simulink model "KALM_filter_DTC_6Sector"  (R2018a)
settings: Solver=ode45  StartTime=0.0  StopTime=6  RelTol=1e-3
values from neighbouring files (symbols this model uses):
  Ah = [0 0 0 0;0 0 0 0;0 1/(Ls*segma) 0 -1;-1/(Ls*segma) 0 1 0]    [Untitled.m]
  Ak = [0 0 -Rs 0; 0 0 0 -Rs; 1/(Tr*Ls*segma) 0 -(1/Ts+1/Tr)/segma 0;     0 1/(Tr*Ls*segma) 0 -(1/Ts+1/Tr)/segma ]    [Untitled.m]
  B = [1 0 1/(Ls*segma) 0;0 1 0 1/(Ls*segma)]'    [Untitled.m]
  J = 0.031    [Untitled.m]
  p = 2    [Untitled.m]
undefined symbols (not defined in the file or in its folder): sigbuilder_block
libraries: powerlib x11, simulink_need_slupdate x1, re_lib x1, powerlib_meascontrol x1
settings Model: Creator=Dell  LastModifiedBy=Dell

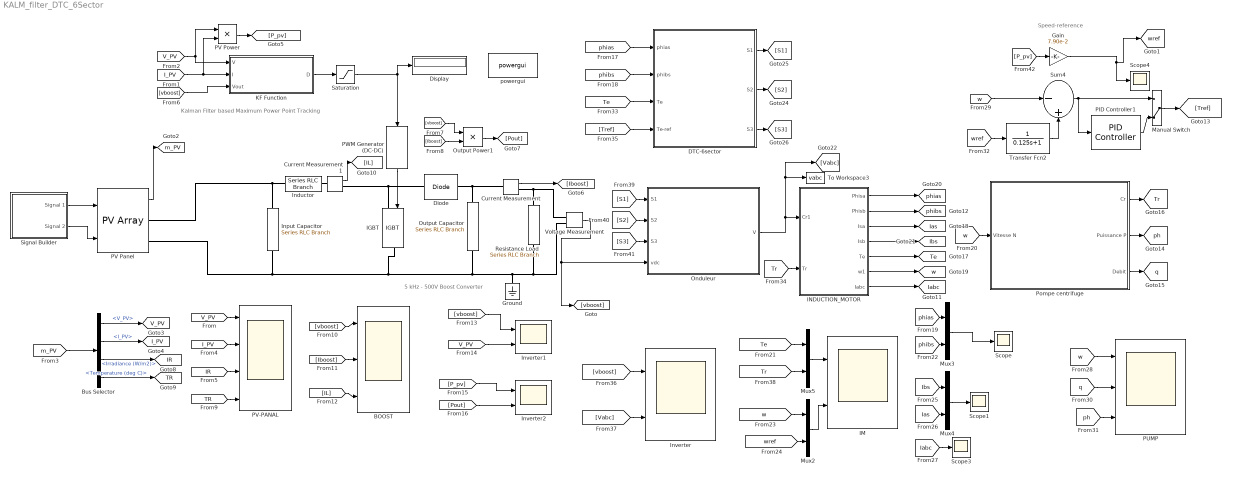
== system KALM_filter_DTC_6Sector ==
  note: 5 kHz - 500V
      | Boost Converter
  note: Kalman Filter based Maximum Power Point Tracking
  note: Speed-reference
  " Resistance Load      " : powerlib/Elements/Series RLC Branch  LConnTagsString=__new0  RConnTagsString=__new0  BranchType=R  Resistance=100  Inductance=1e-3  SetiL0=off  InitialCurrent=0  Capacitance=1e-6  Setx0=off  InitialVoltage=0  Measurements=None
  " Output Capacitor   " : powerlib/Elements/Series RLC Branch  LConnTagsString=__new0  RConnTagsString=__new0  BranchType=C  Resistance=1  Inductance=1e-3  SetiL0=off  InitialCurrent=0  Capacitance=100e-6  Setx0=off  InitialVoltage=0  Measurements=None
  BOOST : Scope  NumInputPorts=3
  Bus Selector : BusSelector  OutputSignals=V_PV,I_PV,Irradiance (W/m2),Temperature (deg C)
  Current Measurement : powerlib/Measurements/Current Measurement  PhasorSimulation=off  OutputType=Complex  PSBequivalent=0
  Current Measurement1 : powerlib/Measurements/Current Measurement  PhasorSimulation=off  OutputType=Complex  PSBequivalent=0
  DTC-6sector : Subsystem
  Diode : powerlib/Power Electronics/Diode  Ron=0.001  Lon=0  Vf=0.8  IC=0  UseSnubber=off  Rs=500  Cs=250e-9  Measurements=off
  Display : Display
  Gain : Gain  Gain=7.90e-2
  Ground : powerlib/Elements/Ground  LConnTagsString=a
  "IGBT  " : powerlib/Power Electronics/IGBT  Ron=0.001  Lon=0  Vf=1  Tf=1e-6  Tt=2e-6  IC=0  Rs=1e5  Cs=inf  Measurements=off
  IM : Scope  NumInputPorts=2
  INDUCTION_MOTOR : Subsystem  mask(Moteur Asynchrone){}
  "Inductor " : powerlib/Elements/Series RLC Branch  LConnTagsString=__new0  RConnTagsString=__new0  BranchType=L  Resistance=0.005  Inductance=3e-3  SetiL0=off  InitialCurrent=0  Capacitance=1e-6  Setx0=off  InitialVoltage=0  Measurements=None
  "Input Capacitor " : powerlib/Elements/Series RLC Branch  LConnTagsString=__new0  RConnTagsString=__new0  BranchType=C  Resistance=1  Inductance=1e-3  SetiL0=off  InitialCurrent=0  Capacitance=100e-6  Setx0=off  InitialVoltage=0  Measurements=None
  Inverter : Scope  NumInputPorts=2
  Inverter1 : Scope  NumInputPorts=2
  Inverter2 : Scope  NumInputPorts=2
  KF Function : MATLAB Function  TreatAsAtomicUnit=on
  Manual Switch : ManualSwitch  CurrentSetting=0
  Mux{2..5} (4 alike) : Mux  Inputs=2
  Onduleur : Subsystem
      mask Display: disp('Onduleur')
  Output Power1 : Product
  PID Controller1 : simulink_need_slupdate/PID Controller  P=4  I=35  D=0
      settings: SourceProductName=Simulink
  PUMP : Scope  NumInputPorts=3
  PV Panel : re_lib/Solar/PV Array  Npar=1  Nser=8  PlotType=array @ 25 deg.C & specified irradiances  S_vec="[800  900 1000   ]"  Temp_C_vec="[ 45 25  ]"  ModuleName=China Sunergy (Nanjing) SST235-60P  PlotWhenSelected=off  Pm=235.024  Ncell=60  Voc=36.8  Isc=8.54  Vm=29.6  Im=7.94  beta_Voc_pc=-0.37  alpha_Isc_pc=0.06  beta_Voc=-0.13616  alpha_Isc=0.005124  IL=8.5548  I0=4.0556e-10  nI=1.0052  Rsh=194.4803  Rs=0.33595  BAL=off  Tc=1e-6  Tfilter=1e-5
      settings: AttributesFormatString=|
      | %<ModuleName>
      | %<Nser>-module string
      | %<Npar> parallel strings
  PV Power : Product
  PV-PANAL : Scope  NumInputPorts=4
  PWM Generator (DC-DC) : powerlib_meascontrol/Pulse & Signal Generators/PWM Generator (DC-DC)  Fsw=5000  Ts=1e-6
  Pompe centrifuge : Subsystem
  "Saturation " : Saturate  UpperLimit=1  LowerLimit=0
  Scope{,1,3..4} (4 alike) : Scope
  Signal Builder : Subsystem  Tag=STV Subsys  LoadFcn=sigbuilder_block('load');  StartFcn=sigbuilder_block('start');  StopFcn=sigbuilder_block('stop');  ClipboardFcn=sigbuilder_block('clipboard');  mask(Sigbuilder block){tuvar=[0:10]}
      mask help: Simulink:masks:SigbuilderBlock_MD
      mask init:
      | if ~strcmp(get_param(bdroot(gcbh),'SimulationStatus'),'stopped') tuvar = sigbuilder_block('maskInit'); end
      settings: CopyFcn=sigbuilder_block('copy');  DeleteFcn=sigbuilder_block('delete');  ModelCloseFcn=sigbuilder_block('modelClose');  PreSaveFcn=sigbuilder_block('preSave');  PauseFcn=sigbuilder_block('pause');  ContinueFcn=sigbuilder_block('continue');  NameChangeFcn=sigbuilder_block('namechange');  OpenFcn=sigbuilder_block('open',[257.25 132.75 550.5 359.25 ]);  CloseFcn=sigbuilder_block('close');
      mask Display: plot(0, 0, 100, 100,[2, 2, 32, 32, 2], [68, 8, 8, 68, 68],[32, 2], [38, 38], [32, 19, 2],[53, 60, 44], [32, 17, 17, 2],[16, 16, 31, 31]);txt = getActiveGroup(gcbh);text(2, 100, txt,'verticalAlignment', 'top');
  Sum4 : Sum  Inputs=|-+  SampleTime=0.00001
  To Workspace3 : ToWorkspace  VariableName=vabc  SampleTime=-1
  Transfer Fcn2 : TransferFcn  Denominator=[0.125 1]
  Voltage Measurement : powerlib/Measurements/Voltage Measurement  PhasorSimulation=off  OutputType=Complex  PSBequivalent=0
  powergui : powerlib/powergui  Priority=1  SimulationMode=Discrete  SampleTime=1e-6  frequency=60  Iterations=50  frequencyindice=0  Pbase=100e6  ErrMax=1e-4  UnitsV=kV  UnitsW=MW  buscounter=0  FunctionMessages=off  echomessages=off  EnableUseOfTLC=off  CurrentSourceSwitches=off  DisableSnubberDevices=off  DisableRonSwitches=off  DisableVfSwitches=off  DisplayEquations=off  SolverType=Tustin/Backward Euler (TBE)  Interpol=off  ExternalGateDelay=off  methode=off  Ts=100  x0status=blocks  SPID=on  SwTol=0  HookPort=off  RestoreLinks=warning  ResistiveCurrentMeasurement=off  Frange=[0:2:500]  Ylog=off  Xlog=on  ShowGrid=off  save=off  variable=ZData  structure=0  ZoomFFT=off  StartTime=0.0  cycles=1  DisplayStyle=1  fundamental=60  FreqAxis=off  MaxFrequency=1000  frequencyindicesteady=1  RmsSteady=1  display=off
  tag scope: IR=global, I_PV=global, Iabc=global, Ias=global, Ibs=global, TR=global, Te=global, Tr=global, V_PV=global, m_PV=global, ph=global, phias=global, phibs=global, q=global, w=global, wref=global
  wires:
  [w] -> PUMP/1
  [IL] -> BOOST/3
  [q] -> PUMP/2
  [w] -> Sum4/1
  [vboost] -> Inverter1/1
  Mux4/1 -> Scope1/1
  [S1] -> Onduleur/1(S1)
  "Saturation "/1 -> Display/1, PWM Generator (DC-DC)/1
  [S3] -> Onduleur/3(S3)
  [phibs] -> DTC-6sector/2(phibs)
  [ph] -> PUMP/3
  [Ias] -> Mux4/2
  DTC-6sector/1(S1) -> [S1]
  INDUCTION_MOTOR/7(Iabc) -> [Iabc]
  Current Measurement1/1 -> [IL]
  Mux5/1 -> IM/1
  [V_PV] -> PV Power/1, KF Function/1(V)
  Signal Builder/1(Signal 1) -> PV Panel/1
  [S2] -> Onduleur/2(S2)
  Bus Selector/1 -> [V_PV]  "<V_PV>"
  INDUCTION_MOTOR/5(Te) -> [Te]
  Pompe centrifuge/3(Debit) -> [q]
  [Pout] -> Inverter2/2
  [Te] -> Mux5/1
  INDUCTION_MOTOR/6(w1) -> [w]
  [Te] -> DTC-6sector/3(Te)
  [w] -> Pompe centrifuge/1(Vitesse N)
  [wref] -> Mux2/2
  [vboost] -> Inverter/1
  Sum4/1 -> Manual Switch/1, PID Controller1/1
  Signal Builder/2(Signal 2) -> PV Panel/2
  [phias] -> DTC-6sector/1(phias)
  [phias] -> Mux3/1
  Manual Switch/1 -> [Tref]
  [w] -> Mux2/1
  [Vabc] -> Inverter/2
  [Tr] -> Mux5/2
  INDUCTION_MOTOR/1(Phisa) -> [phias]
  [Tref] -> DTC-6sector/4(Te-ref)
  [Ibs] -> Mux4/1
  [vboost] -> KF Function/3(Vout)
  [m_PV] -> Bus Selector/1
  Bus Selector/3 -> [IR]  "<Irradiance (W/m2)>"
  [vboost] -> BOOST/1
  [V_PV] -> Inverter1/2
  Bus Selector/4 -> [TR]  "<Temperature (deg C)>"
  [phibs] -> Mux3/2
  [Iboost] -> BOOST/2
  INDUCTION_MOTOR/3(Isa) -> [Ias]
  [vboost] -> Output Power1/1
  PV Power/1 -> [P_pv]
  PWM Generator (DC-DC)/1 -> "IGBT  "/1
  Mux2/1 -> IM/2
  Output Power1/1 -> [Pout]
  DTC-6sector/3(S3) -> [S3]
  [Iboost] -> Output Power1/2
  KF Function/1(D) -> "Saturation "/1
  INDUCTION_MOTOR/2(Phisb) -> [phibs]
  [I_PV] -> PV-PANAL/2
  Voltage Measurement/1 -> Onduleur/4(vdc), [vboost]
  [P_pv] -> Inverter2/1
  Mux3/1 -> Scope/1
  [TR] -> PV-PANAL/4
  [Iabc] -> Scope3/1
  Pompe centrifuge/1(Cr) -> [Tr]
  [Tr] -> INDUCTION_MOTOR/2(Tr)
  Transfer Fcn2/1 -> Sum4/2
  PV Panel/1 -> [m_PV]
  DTC-6sector/2(S2) -> [S2]
  Bus Selector/2 -> [I_PV]  "<I_PV>"
  Pompe centrifuge/2("Puissance P ") -> [ph]
  INDUCTION_MOTOR/4(Isb) -> [Ibs]
  [wref] -> Transfer Fcn2/1
  Onduleur/1(V) -> INDUCTION_MOTOR/1(Cr1), [Vabc], To Workspace3/1
  [V_PV] -> PV-PANAL/1
  [IR] -> PV-PANAL/3
  Current Measurement/1 -> [Iboost]
  PID Controller1/1 -> Manual Switch/2
  [I_PV] -> PV Power/2, KF Function/2(I)
  [P_pv] -> Gain/1
  Gain/1 -> Scope4/1, [wref]
  connections:
  Ground/LConn1 -- PV Panel/RConn2 -- "Input Capacitor "/RConn1 -- "IGBT  "/RConn1 -- " Output Capacitor   "/RConn1 -- " Resistance Load      "/RConn1 -- Voltage Measurement/LConn2
  " Output Capacitor   "/LConn1 -- Diode/RConn1 -- Current Measurement/LConn1
  "Input Capacitor "/LConn1 -- PV Panel/RConn1 -- "Inductor "/LConn1
  "IGBT  "/LConn1 -- Diode/LConn1 -- Current Measurement1/RConn1
  " Resistance Load      "/LConn1 -- Current Measurement/RConn1 -- Voltage Measurement/LConn1
  Current Measurement1/LConn1 -- "Inductor "/RConn1

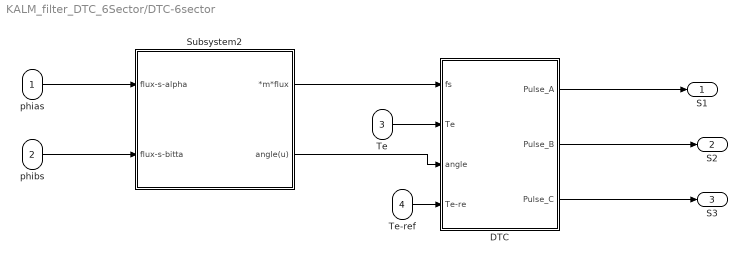
== system KALM_filter_DTC_6Sector/DTC-6sector ==
  phias : Inport
  phibs : Inport  Port=2
  Te : Inport  Port=3
  Te-ref : Inport  Port=4
  DTC : Subsystem
  Subsystem2 : Subsystem
  S1 : Outport
  S2 : Outport  Port=2
  S3 : Outport  Port=3
  wires:
  Te/1 -> DTC/2(Te)
  Subsystem2/1(*m*flux) -> DTC/1(fs)
  DTC/2(Pulse_B) -> S2/1
  Subsystem2/2(angle(u)) -> DTC/3(angle)
  DTC/1(Pulse_A) -> S1/1
  Te-ref/1 -> DTC/4(Te-re)
  DTC/3(Pulse_C) -> S3/1
  phibs/1 -> Subsystem2/2(flux-s-bitta)
  phias/1 -> Subsystem2/1(flux-s-alpha)

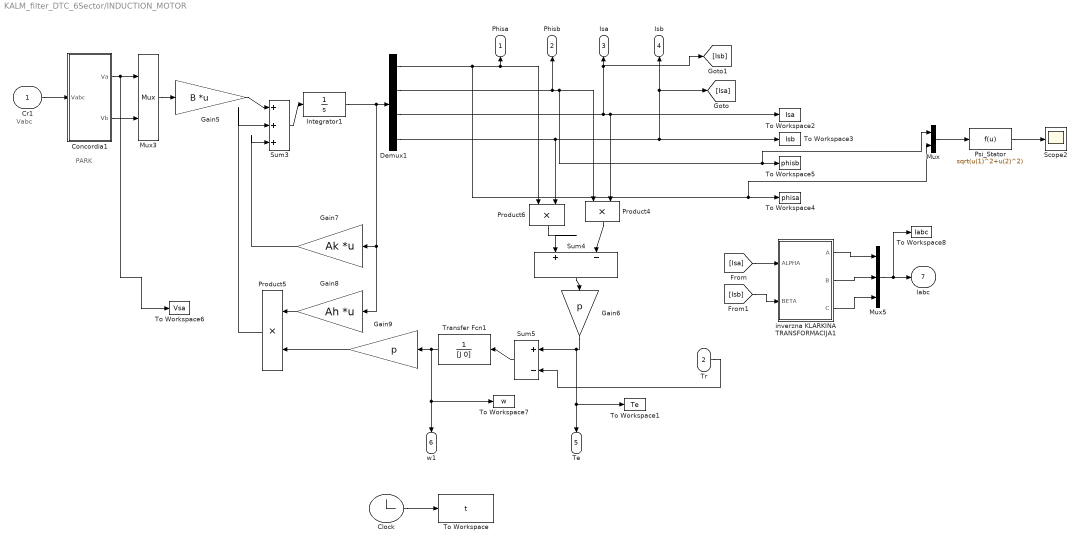
== system KALM_filter_DTC_6Sector/INDUCTION_MOTOR ==
  note: Vabc
  note: PARK
  Cr1 : Inport
  Tr : Inport  Port=2
  Clock : Clock
  Concordia1 : Subsystem
  Demux1 : Demux
  Gain5 : Gain  Gain=B  Multiplication=Matrix(K*u) (u vector)  SampleTime=0.00001
  Gain6 : Gain  Gain=p  SampleTime=0.00001
  Gain7 : Gain  Gain=Ak  Multiplication=Matrix(K*u)  SampleTime=0.00001
  Gain8 : Gain  Gain=Ah  Multiplication=Matrix(K*u)  SampleTime=0.00001
  Gain9 : Gain  Gain=p  SampleTime=0.00001
  Integrator1 : Integrator
  Mux : Mux  Inputs=2
  Mux3 : Mux  Inputs=2
  Mux5 : Mux  Inputs=3
  Product4 : Product  SampleTime=0.00001  RndMeth=Zero
  Product5 : Product  SampleTime=0.00001  RndMeth=Zero
  Product6 : Product  SampleTime=0.00001  RndMeth=Zero
  Psi_Stator : Fcn  Expr=sqrt(u(1)^2+u(2)^2)
  Scope2 : Scope
  Sum3 : Sum  Inputs=|+++  SampleTime=0.00001
  Sum4 : Sum  Inputs=|+-  SampleTime=0.00001
  Sum5 : Sum  Inputs=|+-  SampleTime=0.00001
  To Workspace : ToWorkspace  VariableName=t  SampleTime=0.00001
  To Workspace1 : ToWorkspace  VariableName=Te  SampleTime=-1
  To Workspace2 : ToWorkspace  VariableName=Isa  SampleTime=-1
  To Workspace3 : ToWorkspace  VariableName=Isb  SampleTime=-1
  To Workspace4 : ToWorkspace  VariableName=phisa  SampleTime=-1
  To Workspace5 : ToWorkspace  VariableName=phisb  SampleTime=-1
  To Workspace6 : ToWorkspace  VariableName=Vsa  SampleTime=-1
  To Workspace7 : ToWorkspace  VariableName=w  SampleTime=-1
  To Workspace8 : ToWorkspace  VariableName=Iabc  SampleTime=-1
  Transfer Fcn1 : TransferFcn  Denominator=[J 0]
  inverzna KLARKINA TRANSFORMACIJA1 : Subsystem
  Phisa : Outport
  Phisb : Outport  Port=2
  Isa : Outport  Port=3
  Isb : Outport  Port=4
  Te : Outport  Port=5
  w1 : Outport  Port=6
  Iabc : Outport  Port=7
  wires:
  Gain5/1 -> Sum3/1
  Sum5/1 -> Transfer Fcn1/1
  Gain8/1 -> Product5/1
  Sum3/1 -> Integrator1/1
  Integrator1/1 -> Demux1/1, Gain8/1, Gain7/1
  Clock/1 -> To Workspace/1
  Mux3/1 -> Gain5/1
  Transfer Fcn1/1 -> Gain9/1, w1/1, To Workspace7/1
  Demux1/3 -> Product4/2, To Workspace2/1, [Isb], Isa/1
  Demux1/4 -> Product6/2, Isb/1, [Isa], To Workspace3/1
  Gain6/1 -> Sum5/1, Te/1, To Workspace1/1
  Sum4/1 -> Gain6/1
  Product5/1 -> Sum3/2
  Gain7/1 -> Sum3/3
  Concordia1/2(Vb) -> Mux3/2
  Concordia1/1(Va) -> Mux3/1, To Workspace6/1
  Cr1/1 -> Concordia1/1(Vabc)
  Gain9/1 -> Product5/2
  Product6/1 -> Sum4/1
  Product4/1 -> Sum4/2
  inverzna KLARKINA TRANSFORMACIJA1/1(A) -> Mux5/1
  inverzna KLARKINA TRANSFORMACIJA1/2(B) -> Mux5/2
  Mux5/1 -> To Workspace8/1, Iabc/1
  [Isa] -> inverzna KLARKINA TRANSFORMACIJA1/1(ALPHA)
  [Isb] -> inverzna KLARKINA TRANSFORMACIJA1/2(BETA)
  inverzna KLARKINA TRANSFORMACIJA1/3(C) -> Mux5/3
  Tr/1 -> Sum5/2
  Psi_Stator/1 -> Scope2/1
  Demux1/1 -> Phisa/1, Product6/1, Mux/2, To Workspace4/1
  Mux/1 -> Psi_Stator/1
  Demux1/2 -> Phisb/1, Product4/1, Mux/1, To Workspace5/1

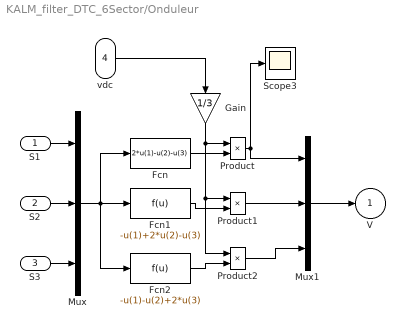
== system KALM_filter_DTC_6Sector/Onduleur ==
  S1 : Inport
  S2 : Inport  Port=2
  S3 : Inport  Port=3
  vdc : Inport  Port=4
  Fcn : Fcn  Expr=2*u(1)-u(2)-u(3)
  Fcn1 : Fcn  Expr=-u(1)+2*u(2)-u(3)
  Fcn2 : Fcn  Expr=-u(1)-u(2)+2*u(3)
  Gain : Gain  Gain=1/3  SaturateOnIntegerOverflow=on  OutDataTypeStr=Inherit: Same as input  ParamDataTypeStr=Inherit: Same as input
  Mux : Mux  Inputs=3
  Mux1 : Mux  Inputs=3
  Product : Product  SaturateOnIntegerOverflow=on  OutDataTypeStr=Inherit: Same as first input
  Product1 : Product  SaturateOnIntegerOverflow=on  OutDataTypeStr=Inherit: Same as first input
  Product2 : Product  SaturateOnIntegerOverflow=on  OutDataTypeStr=Inherit: Same as first input
  Scope3 : Scope
  V : Outport
  wires:
  Product2/1 -> Mux1/3
  Product1/1 -> Mux1/2
  Product/1 -> Mux1/1, Scope3/1
  Gain/1 -> Product2/1, Product1/1, Product/1
  vdc/1 -> Gain/1
  Fcn2/1 -> Product2/2
  Fcn1/1 -> Product1/2
  Fcn/1 -> Product/2
  Mux/1 -> Fcn1/1, Fcn2/1, Fcn/1
  S1/1 -> Mux/1
  S2/1 -> Mux/2
  S3/1 -> Mux/3
  Mux1/1 -> V/1

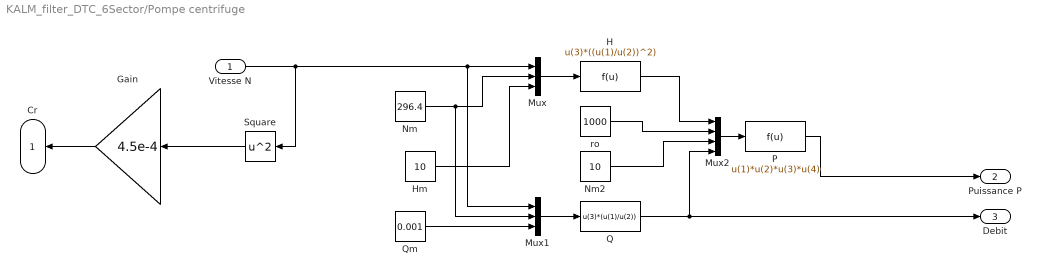
== system KALM_filter_DTC_6Sector/Pompe centrifuge ==
  Vitesse N : Inport
  Gain : Gain  Gain=4.5e-4
  H : Fcn  Expr=u(3)*((u(1)/u(2))^2)
  Hm : Constant  Value=10
  Mux : Mux  Inputs=3
  Mux1 : Mux  Inputs=3
  Mux2 : Mux
  Nm : Constant  Value=296.4
  Nm2 : Constant  Value=10
  "P " : Fcn  Expr=u(1)*u(2)*u(3)*u(4)
  Q : Fcn  Expr=u(3)*(u(1)/u(2))
  Qm : Constant  Value=0.001
  Square : Math  Operator=square  RndMeth=Zero  SaturateOnIntegerOverflow=on
  ro : Constant  Value=1000
  Cr : Outport
  "Puissance P " : Outport  Port=2
  Debit : Outport  Port=3
  wires:
  Square/1 -> Gain/1
  Gain/1 -> Cr/1
  "P "/1 -> "Puissance P "/1
  ro/1 -> Mux2/2
  Qm/1 -> Mux1/3
  Q/1 -> Debit/1, Mux2/4
  Mux2/1 -> "P "/1
  Mux/1 -> H/1
  Nm2/1 -> Mux2/3
  Mux1/1 -> Q/1
  Vitesse N/1 -> Square/1, Mux1/1, Mux/1
  H/1 -> Mux2/1
  Hm/1 -> Mux/3
  Nm/1 -> Mux1/2, Mux/2

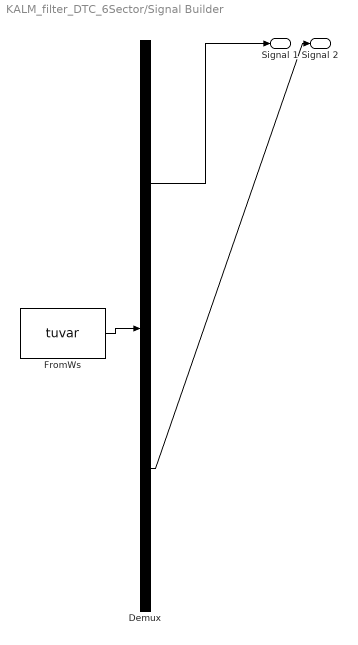
== system KALM_filter_DTC_6Sector/Signal Builder ==
  Demux : Demux  Tag=STV Demux  Outputs=2
  FromWs : FromWorkspace  Tag=STV FromWs  VariableName=tuvar  SampleTime=0
      SigBuilderData=|
      | common.afterFinalStr = 'Extrapolate'
      | common.sampleTime = 0
      | dataSet.timeRange = [0 6]
      | dataSet.name = 'Group 1'
      | sbobj.Groups.Name = 'Group 1'
      | sbobj.Groups.Signals(1).Name = 'Signal 1'
      | sbobj.Groups.Signals(1).XData = [0 1 1 2 2 3 3 4 4 5 5 6]
      | sbobj.Groups.Signals(1).YData = [600 600 800 800 1000 1000 805 800 700 700 600 600]
      | sbobj.Groups.Signals(2).Name = 'Signal 2'
      | sbobj.Groups.Signals(2).XData = [0 6]
      | sbobj.Groups.Signals(2).YData = [25 25]
      | sbobj.Groups.TimeRange = [0 6]
  Signal 1 : Outport  Tag=STV Outport
  Signal 2 : Outport  Tag=STV Outport  Port=2
  wires:
  Demux/1 -> Signal 1/1
  FromWs/1 -> Demux/1
  Demux/2 -> Signal 2/1

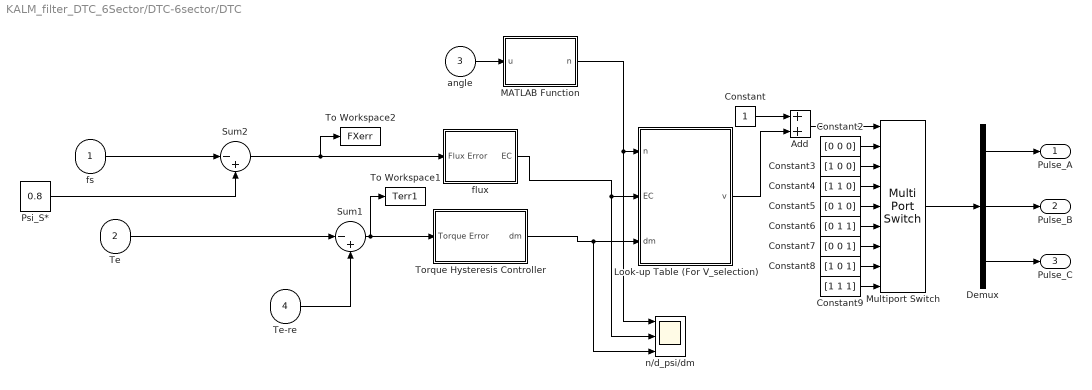
== system KALM_filter_DTC_6Sector/DTC-6sector/DTC ==
  fs : Inport
  Te : Inport  Port=2
  angle : Inport  Port=3
  Te-re : Inport  Port=4
  Add : Sum
  Constant : Constant
  Constant2 : Constant  Value=[0 0 0]
  Constant3 : Constant  Value=[1 0 0]
  Constant4 : Constant  Value=[1 1 0]
  Constant5 : Constant  Value=[0 1 0]
  Constant6 : Constant  Value=[0 1 1]
  Constant7 : Constant  Value=[0 0 1]
  Constant8 : Constant  Value=[1 0 1]
  Constant9 : Constant  Value=[1 1 1]
  Demux : Demux  Outputs=3
  Look-up Table (For V_selection) : MATLAB Function  TreatAsAtomicUnit=on
  MATLAB Function : MATLAB Function  TreatAsAtomicUnit=on
  Multiport Switch : MultiPortSwitch  Inputs=8
  Psi_S* : Constant  Value=0.8
  Sum1 : Sum  Inputs=|-+
  Sum2 : Sum  Inputs=|-+
  To Workspace1 : ToWorkspace  VariableName=Terr1  SampleTime=-1
  To Workspace2 : ToWorkspace  VariableName=FXerr  SampleTime=-1
  Torque Hysteresis Controller : Subsystem
  flux : Subsystem
  n/d_psi/dm : Scope  NumInputPorts=3
  Pulse_A : Outport
  Pulse_B : Outport  Port=2
  Pulse_C : Outport  Port=3
  wires:
  fs/1 -> Sum2/1
  MATLAB Function/1(n) -> Look-up Table (For V_selection)/1(n), n/d_psi/dm/1
  Torque Hysteresis Controller/1(dm) -> Look-up Table (For V_selection)/3(dm), n/d_psi/dm/3
  Psi_S*/1 -> Sum2/2
  Add/1 -> Multiport Switch/1
  Te/1 -> Sum1/1
  Constant9/1 -> Multiport Switch/9
  Constant6/1 -> Multiport Switch/6
  Constant2/1 -> Multiport Switch/2
  Constant3/1 -> Multiport Switch/3
  Constant5/1 -> Multiport Switch/5
  Demux/3 -> Pulse_C/1
  Constant8/1 -> Multiport Switch/8
  Look-up Table (For V_selection)/1(v) -> Add/2
  Constant/1 -> Add/1
  Demux/1 -> Pulse_A/1
  Demux/2 -> Pulse_B/1
  Constant7/1 -> Multiport Switch/7
  Constant4/1 -> Multiport Switch/4
  Multiport Switch/1 -> Demux/1
  flux/1(EC) -> Look-up Table (For V_selection)/2(EC), n/d_psi/dm/2
  Sum2/1 -> To Workspace2/1, flux/1(Flux Error)
  angle/1 -> MATLAB Function/1(u)
  Sum1/1 -> To Workspace1/1, Torque Hysteresis Controller/1(Torque Error)
  Te-re/1 -> Sum1/2

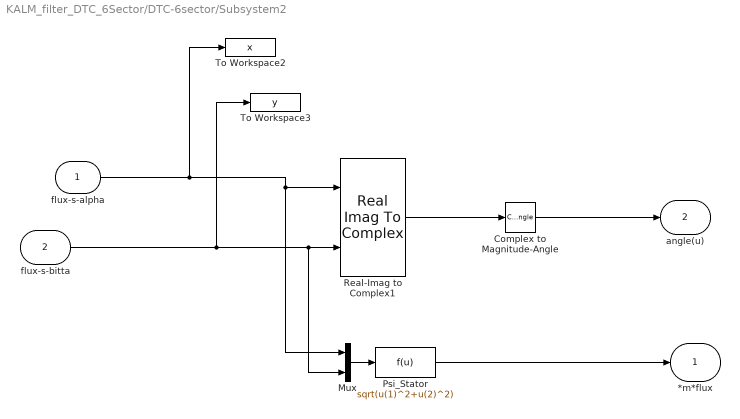
== system KALM_filter_DTC_6Sector/DTC-6sector/Subsystem2 ==
  flux-s-alpha : Inport
  flux-s-bitta : Inport  Port=2
  Complex to Magnitude-Angle : ComplexToMagnitudeAngle  Output=Angle
  Mux : Mux  Inputs=2
  Psi_Stator : Fcn  Expr=sqrt(u(1)^2+u(2)^2)
  Real-Imag to Complex1 : RealImagToComplex  SampleTime=0.00001
  To Workspace2 : ToWorkspace  VariableName=x  SampleTime=-1
  To Workspace3 : ToWorkspace  VariableName=y  SampleTime=-1
  *m*flux : Outport
  angle(u) : Outport  Port=2
  wires:
  Real-Imag to Complex1/1 -> Complex to Magnitude-Angle/1
  Complex to Magnitude-Angle/1 -> angle(u)/1
  Mux/1 -> Psi_Stator/1
  Psi_Stator/1 -> *m*flux/1
  flux-s-alpha/1 -> To Workspace2/1, Mux/1, Real-Imag to Complex1/1
  flux-s-bitta/1 -> Mux/2, Real-Imag to Complex1/2, To Workspace3/1

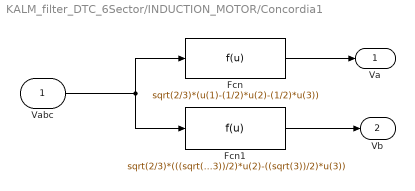
== system KALM_filter_DTC_6Sector/INDUCTION_MOTOR/Concordia1 ==
  Vabc : Inport
  Fcn : Fcn  Expr=sqrt(2/3)*(u(1)-(1/2)*u(2)-(1/2)*u(3))  SampleTime=0.00001
  Fcn1 : Fcn  Expr=sqrt(2/3)*(((sqrt(3))/2)*u(2)-((sqrt(3))/2)*u(3))  SampleTime=0.00001
  Va : Outport
  Vb : Outport  Port=2
  wires:
  Fcn/1 -> Va/1
  Fcn1/1 -> Vb/1
  Vabc/1 -> Fcn/1, Fcn1/1

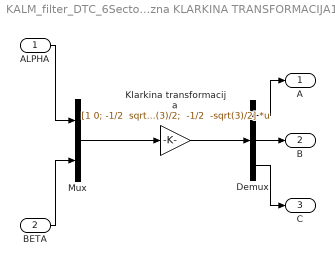
== system KALM_filter_DTC_6Sector/INDUCTION_MOTOR/inverzna KLARKINA TRANSFORMACIJA1 ==
  ALPHA : Inport
  BETA : Inport  Port=2
  Demux : Demux  Outputs=3
  Klarkina transformacija : Gain  Gain="[1 0; -1/2  sqrt(3)/2;  -1/2  -sqrt(3)/2]"  Multiplication=Matrix(K*u)
  Mux : Mux  Inputs=2
  A : Outport
  B : Outport  Port=2
  C : Outport  Port=3
  wires:
  Demux/2 -> B/1
  Demux/1 -> A/1
  ALPHA/1 -> Mux/1
  BETA/1 -> Mux/2
  Klarkina transformacija/1 -> Demux/1
  Mux/1 -> Klarkina transformacija/1
  Demux/3 -> C/1

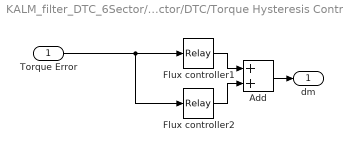
== system KALM_filter_DTC_6Sector/DTC-6sector/DTC/Torque Hysteresis Controller ==
  Torque Error : Inport
  Add : Sum
  Flux controller1 : Relay  OnSwitchValue=0.002  OffSwitchValue=0
  Flux controller2 : Relay  OnSwitchValue=0  OffSwitchValue=-0.002  OnOutputValue=0  OffOutputValue=-1
  dm : Outport
  wires:
  Add/1 -> dm/1
  Flux controller2/1 -> Add/2
  Flux controller1/1 -> Add/1
  Torque Error/1 -> Flux controller2/1, Flux controller1/1

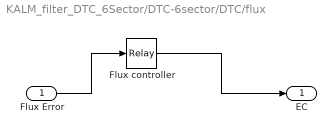
== system KALM_filter_DTC_6Sector/DTC-6sector/DTC/flux ==
  Flux Error : Inport
  Flux controller : Relay  OnSwitchValue=0.0002  OffSwitchValue=-0.0002
  EC : Outport
  wires:
  Flux Error/1 -> Flux controller/1
  Flux controller/1 -> EC/1

== matlab function KALM_filter_DTC_6Sector/DTC-6sector/DTC/Look-up Table (For V_selection) ==
  data: n input; EC input; v output; dm input
function v=V_selection(n,EC,dm)
v=0;
%SECTOR 1 :
if(n==1)&&(EC==1)&&(dm==1)
    v=2;
end
if(n==1)&&(EC==1)&&(dm==0)
    v=7;
end
if(n==1)&&(EC==1)&&(dm==-1)
    v=6;
end
if(n==1)&&(EC==0)&&(dm==1)
    v=3;
end
if(n==1)&&(EC==0)&&(dm==0)
    v=0;
end
if(n==1)&&(EC==0)&&(dm==-1)
    v=5;
end
%SECTOR 2 :
if(n==2)&&(EC==1)&&(dm==1)
    v=3;
end
if(n==2)&&(EC==1)&&(dm==0)
    v=0;
end
if(n==2)&&(EC==1)&&(dm==-1)
    v=1;
end
if(n==2)&&(EC==0)&&(dm==1)
    v=4;
end
if(n==2)&&(EC==0)&&(dm==0)
    v=7;
end
if(n==2)&&(EC==0)&&(dm==-1)
    v=6;
end
%SECTOR 3 :
if(n==3)&&(EC==1)&&(dm==1)
    v=4;
end
if(n==3)&&(EC==1)&&(dm==0)
    v=7;
end
if(n==3)&&(EC==1)&&(dm==-1)
    v=2;
end
if(n==3)&&(EC==0)&&(dm==1)
    v=5;
end
if(n==3)&&(EC==0)&&(dm==0)
    v=0;
end
if(n==3)&&(EC==0)&&(dm==-1)
    v=1;
end
%SECTOR 4 :
if(n==4)&&(EC==1)&&(dm==1)
    v=5;
end
if(n==4)&&(EC==1)&&(dm==0)
    v=0;
end
if(n==4)&&(EC==1)&&(dm==-1)
    v=3;
end
if(n==4)&&(EC==0)&&(dm==1)
    v=6;
end
if(n==4)&&(EC==0)&&(dm==0)
    v=7;
end
if(n==4)&&(EC==0)&&(dm==-1)
    v=2;
end
%SECTOR 5 :
if(n==5)&&(EC==1)&&(dm==1)
    v=6;
end
if(n==5)&&(EC==1)&&(dm==0)
    v=7;
end
if(n==5)&&(EC==1)&&(dm==-1)
    v=4;
end
if(n==5)&&(EC==0)&&(dm==1)
    v=1;
end
if(n==5)&&(EC==0)&&(dm==0)
    v=0;
end
if(n==5)&&(EC==0)&&(dm==-1)
    v=3;
end
%SECTOR 6 :
if(n==6)&&(EC==1)&&(dm==1)
    v=1;
end
if(n==6)&&(EC==1)&&(dm==0)
    v=0;
end
if(n==6)&&(EC==1)&&(dm==-1)
    v=5;
end
if(n==6)&&(EC==0)&&(dm==1)
    v=2;
end
if(n==6)&&(EC==0)&&(dm==0)
    v=7;
end
if(n==6)&&(EC==0)&&(dm==-1)
    v=4;
end

== matlab function KALM_filter_DTC_6Sector/KF Function ==
  data: V input; D output; I input; Vout input
function D = KalmanFilter(V, I, Vout)

% PARAMETERS DEFINATION
A = 1; %Matrix A
step = 18; %step size
B = step; %Matrix B
C = 1; %Matrix C
Vmpp = 236; %Maximum power point voltage (in volts)
Impp = 7.94; %Maximum power point current (in Amp)
Q = 50; 
R = 50;

% KF PARAMETERS INTIALISATION
%STEP-I
persistent v_k
if isempty(v_k)
    v_k = Vmpp;
end
persistent power_k
if isempty(power_k)
    power_k = Vmpp*Impp;
end
persistent v_k_prev
if isempty(v_k_prev)
    v_k_prev = 0;
end
persistent power_k_prev
if isempty(power_k_prev)
    power_k_prev = 0;
end
persistent h_k
if isempty(h_k)
    h_k = 1;
end

pv_slope = (power_k - power_k_prev)/(v_k - v_k_prev);

%KF IMPLEMENTATION
% STAGE - PREDICTION
%STEP-II: Project the state ahead
v_neg = v_k + step*pv_slope;

%STEP-III: Project the error covariance ahead
h_neg = h_k + Q;

% STAGE - UPDATION
% STEP-IV: Compute the kalman gain
K_ = (h_neg)/(h_neg + R);

% STEP-V: Update estimate with measurement Vout
v = v_neg + K_*(V - v_neg);

% STEP-VI: Update the error covariance
h = (1-K_)*h_neg;

% STEP-VII: Saving for next stage
h_k = h;
v_k_prev = v_k;
power_k_prev = power_k;
v_k = V;
power_k = V*I;

% OUTPUT DUTY CYCLE
D = 1 - (v/Vout);
end

== matlab function KALM_filter_DTC_6Sector/DTC-6sector/DTC/MATLAB Function ==
  data: u input; n output
function n=secteur(u)
n=0;
if(u>=-pi/6)&&(u<pi/6)
    n=1;
end
if(u>=pi/6)&&(u<pi/2)
    n=2;
end
if(u>=pi/2)&&(u<5*pi/6)
    n=3;
end
if(u>=5*pi/6)&&(u<pi)
    n=4;
end
if(u>=-pi)&&(u<-5*pi/6)
    n=4;
end
if(u>=-5*pi/6)&&(u<-pi/2)
    n=5;
end
if(u>=-pi/2)&&(u<-pi/6)
    n=6;
end
